simulink subsystem "EncodersN20"  (R2025a)
settings: Solver=VariableStepAuto  StartTime=0.0  StopTime=10.0  RelTol=1e-3
libraries: arduinosensorlib x4, simulink x1, eeGeneralControl x1
settings Model: Creator=Antonio  LastModifiedBy=aj
settings RTWCC: GPUComputeCapability=3.5

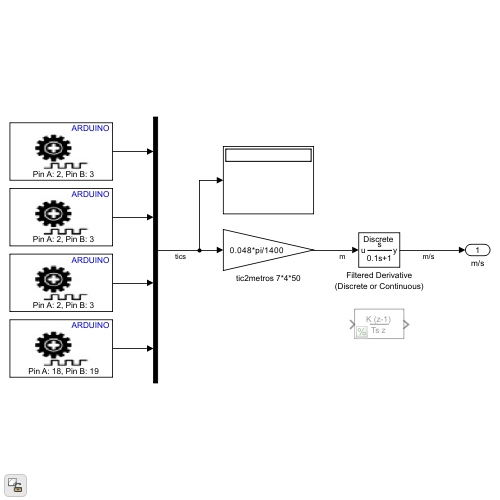
[thumbnail: Simulink's stored preview of the top-level diagram]
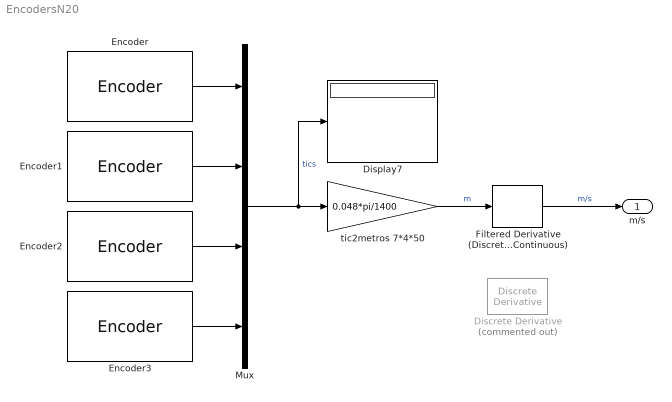
== system EncodersN20 ==
  Discrete Derivative : simulink/Discrete/Discrete Derivative  Commented=on  gainval=1.0  ICPrevScaledInput=0.0  OutMin=[]  OutMax=[]  OutDataType=fixdt(1, 16)  OutScaling=2^-10  DoSatur=off
  Display7 : Display
  Encoder : arduinosensorlib/Encoder  InputA=34  InputB=35  Mode=No reset  SampleTime=-1
  Encoder1 : arduinosensorlib/Encoder  InputA=5  InputB=17  Mode=No reset  SampleTime=-1
  Encoder2 : arduinosensorlib/Encoder  InputA=39  InputB=36  Mode=No reset  SampleTime=-1
  Encoder3 : arduinosensorlib/Encoder  InputA=18  InputB=19  Mode=No reset  SampleTime=-1
  Filtered Derivative (Discrete or Continuous) : eeGeneralControl/Filtered Derivative (Discrete or Continuous)  K=1  T=0.1  B=inf  A=-inf  minRatio=10  init_option=Inherited from block input  x0=0  Ts=-1
      settings: LibrarySourceBlock=|
      | ee_sl_lib/General Control/Filtered Derivative
      | (Discrete or Continuous)
  Mux : Mux
  tic2metros 7*4*50 : Gain  Gain=0.048*pi/1400  OutDataTypeStr=double
  m/s : Outport
  wires:
  Filtered Derivative (Discrete or Continuous)/1 -> m/s/1  "m/s"
  tic2metros 7*4*50/1 -> Filtered Derivative (Discrete or Continuous)/1  "m"
  Mux/1 -> Display7/1, tic2metros 7*4*50/1  "tics"
  Encoder2/1 -> Mux/3
  Encoder/1 -> Mux/1
  Encoder3/1 -> Mux/4
  Encoder1/1 -> Mux/2
